simulink model "Com_hex2num_convert"  (R2017a)
settings: Solver=ode3  StartTime=0.0  StopTime=Inf  FixedStep=0.05  RelTol=1e-3  EnableMultiTasking=on
PostLoadFcn:
  | , if any(exist('dsrtsu_mdlpostloadfcn', 'file') == [2, 3, 6]), try dsrtsu_mdlpostloadfcn('Execute', bdroot); catch fprintf('Error in PostLoadFcn (dsrtsu_mdlpostloadfcn) for model "%s":\n %s\n', bdroot, lasterr); end, end,
undefined symbols (not defined in the file): serial
libraries: instrumentlib x2
settings Model: DSRTSU_INTERNAL_RTI_VER=500  DSRTSU_INTERNAL_RTI_TYPE=rti1401  DSRTSU_INTERNAL_RTIFPGA=90  Creator=Administrator  LastModifiedBy=Administrator
settings DataIOCC: SaveFormat=Array
settings OptimizationCC: BlockReduction=off  OptimizeBlockIOStorage=off  BufferReuse=off  GlobalBufferReuse=off  ExpressionFolding=off  LocalBlockOutputs=off  LifeSpan=inf
settings DebuggingCC: UnderspecifiedInitializationDetection=Classic  MergeDetectMultiDrivingBlocksExec=none  SolverPrmCheckMsg=warning  StateNameClashWarn=warning  SFUnexpectedBacktrackingDiag=warning  SFNoUnconditionalDefaultTransitionDiag=warning  SFExecutionAtInitializationDiag=none
settings HardwareCC: ProdBitPerPointer=32  ProdBitPerSizeT=32  ProdBitPerPtrDiffT=32  ProdLargestAtomicInteger=Integer  ProdEndianess=BigEndian  ProdWordSize=32  ProdHWDeviceType=Custom Processor->Custom  TargetIntDivRoundTo=Zero  TargetEndianess=BigEndian  TargetHWDeviceType=Custom Processor->Custom
settings ModelReferenceCC: PropagateSignalLabelsOutOfModel=off
settings SFSimCC: MATLABDynamicMemAlloc=off
settings RTWCC: SystemTargetFile=rti1005.tlc  MakeCommand=make_rti  TemplateMakefile=rti1005.tmf  Description=dSPACE DS1005 Hardware Platform
settings STFCustomTargetCC: ParMdlRefBuildCompliant=on  GRTInterface=off  SystemTargetFile=rti1005.tlc
settings GRTTargetCC: TargetLangStandard=C89/C90 (ANSI)  CompOptLevelCompliant=off  ConcurrentExecutionCompliant=off  CombineOutputUpdateFcns=off  MatFileLogging=off  CPPClassGenCompliant=off  UseToolchainInfoCompliant=off  ExtModeMexFile=noextcomm
settings ConfigComp: CovMetricSettings=dw  CovHtmlReporting=on  CovSaveCumulativeToWorkspaceVar=on  CovSaveSingleToWorkspaceVar=on  CovExternalEMLEnable=off  CovSFcnEnable=off

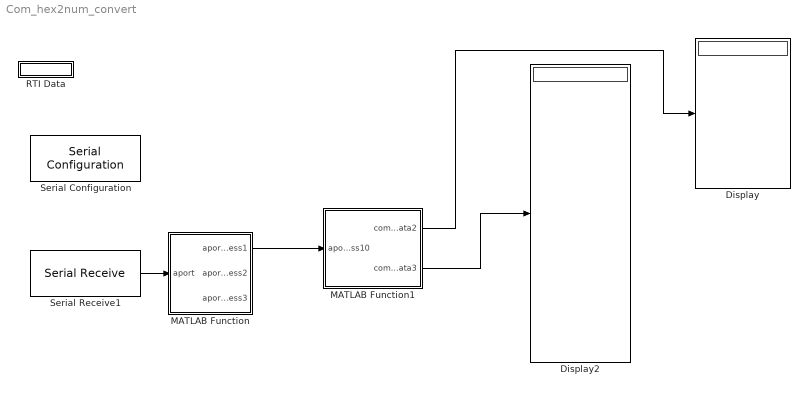
== system Com_hex2num_convert ==
  Display : Display
  Display2 : Display
  MATLAB Function : MATLAB Function  TreatAsAtomicUnit=on
  MATLAB Function1 : MATLAB Function  TreatAsAtomicUnit=on
  RTI Data : Subsystem  Tag=struct('RTIDataServer',struct('RTIDataServerVs','2','RTIModelDescription','struct(''main'',''Com_hex2num_convert'',''sub'',''Com_hex2num_convert'',''isMp'',0)'))  LoadFcn="if exist('rtidc'), try,  rtidc('DataHostBlockClbLoad', gcbh); catch, disp(['Warning: ''LoadFcn'' for RTI Data block failed: ' lasterr]); end, end,"  mask(RTI_DATA_HOST){}
      mask help:
      | RTI Data Block.
      | This block is used by RTI to store internal model-dependent data.
      | Please keep this block on the root level of the model. Deleting this block will result in data loss.
      |
      | NEVER DELETE OR COPY THIS BLOCK!
      settings: CopyFcn="if exist('rtidc'), try,  rtidc('DataHostBlockClbCopy', gcbh); catch, disp(['Warning: ''CopyFcn'' for RTI Data block failed: ' lasterr]); end, end,"  DeleteFcn="if exist('rtidc'), try,  rtidc('DataHostBlockClbDelete', gcbh); catch, disp(['Warning: ''DeleteFcn'' for RTI Data block failed: ' lasterr]); end, end,"  ModelCloseFcn="if exist('rtidc'), try,  rtidc('DataHostBlockClbModelClose', gcbh); catch, disp(['Warning: ''ModelCloseFcn'' for RTI Data block failed: ' lasterr]); end, end,"  PreSaveFcn="if exist('rtidc'), try,  rtidc('DataHostBlockClbPreSave', gcbh); catch, disp(['Warning: ''PreSaveFcn'' for RTI Data block failed: ' lasterr]); end, end,"  PostSaveFcn="if exist('rtidc'), try,  rtidc('DataHostBlockClbPostSave', gcbh); catch, disp(['Warning: ''PostSaveFcn'' for RTI Data block failed: ' lasterr]); end, end,"  NameChangeFcn="if exist('rtidc'), try,  rtidc('DataHostBlockClbNameChange', gcbh); catch, disp(['Warning: ''NameChangeFcn'' for RTI Data block failed: ' lasterr]); end, end,"
      mask Help:
      | RTI Data Block.
      | This block is used by RTI to store internal model-dependent data.
      | Please keep this block on the root level of the model. Deleting this block will result in data loss.
      | 
      | NEVER DELETE OR COPY THIS BLOCK!
      mask Display:
      | text(0.5, 0.5, 'RTI Data', 'HorizontalAlignment', 'center');
      | plot([1 0]);
  Serial Configuration : instrumentlib/Serial Configuration  Priority=-200000  ComPortMenu=<Please select a port...>  ComPort=COM4  ObjConstructor=serial('COM4');  BaudRate=115200  DataBits=8  Parity=none  StopBits=1  FlowControl=none  Timeout=10  ByteOrder=LittleEndian
  Serial Receive1 : instrumentlib/Serial Receive  ComPortMenu=<Please select a port...>  ComPort=COM4  ObjConstructor=serial('COM4');  Terminator=<none>  DataSize="[600    1]"  DataType=uint8  EnableBlockingMode=on  ActionDataUnavailable=Output last received value  CustomValue=0  SampleTime=0.05
  wires:
  Serial Receive1/1 -> MATLAB Function/1(aport)
  MATLAB Function/1(aport_mess1) -> MATLAB Function1/1(aport_mess10)
  MATLAB Function1/2(com_data3) -> Display2/1
  MATLAB Function1/1(com_data2) -> Display/1

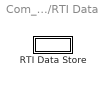
== system Com_hex2num_convert/RTI Data ==
  RTI Data Store : Subsystem  Tag=struct('private',struct('version',struct('dsVer',uint32(2),'dsVerCreation',uint32(2),'RTI',struct('ver','7.1','type','RTI1005')),'access',struct('type','Model','isPerm',1,'created',['10-Nov-2015 11:46:18'],'modified',['27-Sep-2017 17:37:50'],'location','')),'public',struct('main',struct('data',[]),'sub',struct('name','','data',[])))  mask(RTI_DATA_STORE){}
      mask help:
      | RTI Data Store Block. This block is used by RTI to store internal model dependent data. Deleting this block will result in data loss.
      |
      | NEVER DELETE, COPY, OR MODIFY THIS BLOCK!
      mask Help:
      | RTI Data Store Block. This block is used by RTI to store internal model dependent data. Deleting this block will result in data loss.
      | 
      | NEVER DELETE, COPY, OR MODIFY THIS BLOCK!
      mask Display: text(0.5, 0.5, ' ', 'HorizontalAlignment', 'center');

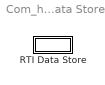
== system Com_hex2num_convert/RTI Data/RTI Data Store ==
  RTI Data Store : Subsystem  mask(RTI_DATA_STORE){}
      mask help:
      | RTI Data Store Block. This block is used by RTI to store internal model dependent data. Deleting this block will result in data loss.
      |
      | NEVER DELETE, COPY, OR MODIFY THIS BLOCK!
      mask Help:
      | RTI Data Store Block. This block is used by RTI to store internal model dependent data. Deleting this block will result in data loss.
      | 
      | NEVER DELETE, COPY, OR MODIFY THIS BLOCK!
      mask Display: text(0.5, 0.5, ' ', 'HorizontalAlignment', 'center');

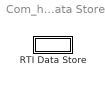
== system Com_hex2num_convert/RTI Data/RTI Data Store/RTI Data Store ==
  RTI Data Store : Subsystem  mask(RTI_DATA_STORE){}
      mask help:
      | RTI Data Store Block. This block is used by RTI to store internal model dependent data. Deleting this block will result in data loss.
      |
      | NEVER DELETE, COPY, OR MODIFY THIS BLOCK!
      mask Help:
      | RTI Data Store Block. This block is used by RTI to store internal model dependent data. Deleting this block will result in data loss.
      | 
      | NEVER DELETE, COPY, OR MODIFY THIS BLOCK!
      mask Display: text(0.5, 0.5, ' ', 'HorizontalAlignment', 'center');

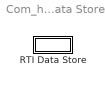
== system Com_hex2num_convert/RTI Data/RTI Data Store/RTI Data Store/RTI Data Store ==
  RTI Data Store : Subsystem  mask(RTI_DATA_STORE){}
      mask help:
      | RTI Data Store Block. This block is used by RTI to store internal model dependent data. Deleting this block will result in data loss.
      |
      | NEVER DELETE, COPY, OR MODIFY THIS BLOCK!
      mask Help:
      | RTI Data Store Block. This block is used by RTI to store internal model dependent data. Deleting this block will result in data loss.
      | 
      | NEVER DELETE, COPY, OR MODIFY THIS BLOCK!
      mask Display: text(0.5, 0.5, ' ', 'HorizontalAlignment', 'center');

== system Com_hex2num_convert/RTI Data/RTI Data Store/RTI Data Store/RTI Data Store/RTI Data Store ==

== matlab function Com_hex2num_convert/MATLAB Function1 ==
  data: aport_mess10 input; com_data2 output; com_data3 output
function [com_data2, com_data3]  = GNSS_data(aport_mess10)
com_data20=zeros(3,1);
com_data30=zeros(16,1);
for i=1
aport_mess1=aport_mess10(i,:);

com_01=aport_mess1(1:4);
com_01=fliplr(com_01);

com_02=(aport_mess1(5:8));  %time seconds
com_02=(dec2hex(fliplr(com_02)));
com_02=[com_02(1,:),com_02(2,:),com_02(3,:),com_02(4,:)];
com_02=hex2dec(com_02);

com_03=(aport_mess1(9:12));  %time microseconds
com_03=(dec2hex(fliplr(com_03)));
com_03=[com_03(1,:),com_03(2,:),com_03(3,:),com_03(4,:)];
com_03=hex2dec(com_03);


com_04=(aport_mess1(13:20));  %纬度  deg
com_04=(dec2hex(fliplr(com_04)));
com_040=[com_04(1,:),com_04(2,:),com_04(3,:),com_04(4,:),com_04(5,:),com_04(6,:),com_04(7,:),com_04(8,:)];
%hex2num(com_042)
com_0410=typecast(uint8((com_040)),'double');
com_041 = com_0410(1,1);
%com_041=com_041*180/pi;

com_05=(aport_mess1(21:28));  %经度 deg
com_05=(dec2hex(fliplr(com_05)));
com_05=[com_05(1,:),com_05(2,:),com_05(3,:),com_05(4,:),com_05(5,:),com_05(6,:),com_05(7,:),com_05(8,:)];
%com_051=[com_05(1,:),com_05(2,:),com_05(3,:),com_05(4,:)]
%com_051=hex2num(com_051);
%com_051=typecast((hex2dec(com_051)),'single')
%com_05=com_05*180/pi;
com_051=0;

com_06=(aport_mess1(29:36));  %高度 m
com_06=(dec2hex(fliplr(com_06)));
com_06=[com_06(1,:),com_06(2,:),com_06(3,:),com_06(4,:),com_06(5,:),com_06(6,:),com_06(7,:),com_06(8,:)];
%com_061=[com_06(1,:),com_06(2,:),com_06(3,:),com_06(4,:)]
%com_061=[com_06(5,:),com_06(6,:),com_06(7,:),com_06(8,:)]
%com_061=hex2num(com_061);
%com_061=typecast((hex2dec(com_061)),'single')
com_061=0;

com_07=(aport_mess1(37:40));  %北向速度 （m/s）
com_07=(dec2hex(fliplr(com_07)));
com_07=[com_07(1,:),com_07(2,:),com_07(3,:),com_07(4,:)];
com_07=typecast(uint32(hex2dec(com_07)),'single');

com_08=(aport_mess1(41:44));  %东向速度 （m/s）
com_08=(dec2hex(fliplr(com_08)));
com_08=[com_08(1,:),com_08(2,:),com_08(3,:),com_08(4,:)];
com_08=typecast(uint32(hex2dec(com_08)),'single');

com_09=(aport_mess1(45:48));  %地向速度 （m/s）
com_09=(dec2hex(fliplr(com_09)));
com_09=[com_09(1,:),com_09(2,:),com_09(3,:),com_09(4,:)];
com_09=typecast(uint32(hex2dec(com_09)),'single');

com_10=(aport_mess1(49:52));  % 载体加速度 X（m/s/s）
com_10=(dec2hex(fliplr(com_10)));
com_10=[com_10(1,:),com_10(2,:),com_10(3,:),com_10(4,:)];
com_10=typecast(uint32(hex2dec(com_10)),'single');

com_11=(aport_mess1(53:56));  % 载体加速度 Y（m/s/s）
com_11=(dec2hex(fliplr(com_11)));
com_11=[com_11(1,:),com_11(2,:),com_11(3,:),com_11(4,:)];
com_11=typecast(uint32(hex2dec(com_11)),'single');

com_12=(aport_mess1(57:60));  % 载体加速度 Z（m/s/s）
com_12=(dec2hex(fliplr(com_12)));
com_12=[com_12(1,:),com_12(2,:),com_12(3,:),com_12(4,:)];
com_12=typecast(uint32(hex2dec(com_12)),'single');

com_13=(aport_mess1(61:64));  % % 重力加速度 （g）
com_13=(dec2hex(fliplr(com_13)));
com_13=[com_13(1,:),com_13(2,:),com_13(3,:),com_13(4,:)];
com_13=typecast(uint32(hex2dec(com_13)),'single');

com_14=(aport_mess1(65:68));  %横滚 （roll  rad）
com_14=(dec2hex(fliplr(com_14)));
com_14=[com_14(1,:),com_14(2,:),com_14(3,:),com_14(4,:)];
com_14=typecast(uint32(hex2dec(com_14)),'single')*180/pi;  % （deg/s）

com_15=(aport_mess1(69:72));   %俯仰 （roll  rad）
com_15=(dec2hex(fliplr(com_15)));
com_15=[com_15(1,:),com_15(2,:),com_15(3,:),com_15(4,:)];
com_15=typecast(uint32(hex2dec(com_15)),'single')*180/pi;  % （deg/s）

com_16=(aport_mess1(73:76));   %航向 （roll  rad）
com_16=(dec2hex(fliplr(com_16)));
com_16=[com_16(1,:),com_16(2,:),com_16(3,:),com_16(4,:)];
com_16=typecast(uint32(hex2dec(com_16)),'single')*180/pi;  % （deg/s）

com_17=(aport_mess1(77:80));  %角速度 X （rad/s）
com_17=(dec2hex(fliplr(com_17)));
com_17=[com_17(1,:),com_17(2,:),com_17(3,:),com_17(4,:)];
com_17=typecast(uint32(hex2dec(com_17)),'single')*180/pi;  %角速度 X （deg/s）

com_18=(aport_mess1(81:84));  %角速度 Y （rad/s）
com_18=(dec2hex(fliplr(com_18)));
com_18=[com_18(1,:),com_18(2,:),com_18(3,:),com_18(4,:)];
com_18=typecast(uint32(hex2dec(com_18)),'single')*180/pi;  %角速度 Y （deg/s）

com_19=(aport_mess1(85:88));  %角速度 Z （rad/s）
com_19=(dec2hex(fliplr(com_19)));
com_19=[com_19(1,:),com_19(2,:),com_19(3,:),com_19(4,:)];
com_19=typecast(uint32(hex2dec(com_19)),'single')*180/pi;  %角速度 Z （deg/s）

com_20=(aport_mess1(89:92));  %纬度标准差（m）
com_20=(dec2hex(fliplr(com_20)));
com_20=[com_20(1,:),com_20(2,:),com_20(3,:),com_20(4,:)];
com_20=typecast(uint32(hex2dec(com_20)),'single');

com_21=(aport_mess1(93:96));  %经度标准差（m）
com_21=(dec2hex(fliplr(com_21)));
com_21=[com_21(1,:),com_21(2,:),com_21(3,:),com_21(4,:)];
com_21=typecast(uint32(hex2dec(com_21)),'single');

com_22=(aport_mess1(97:100));  %高度标准差（m）
com_22=(dec2hex(fliplr(com_22)));
com_22=[com_22(1,:),com_22(2,:),com_22(3,:),com_22(4,:)];
com_22= typecast(uint32(hex2dec(com_22)),'single');

com_data1=[com_01,com_02,com_03]';     %% time 
com_data20(:,i)=[com_041,com_051,com_061]';    
com_data30(:,i)=[com_07,com_08,com_09,...
          com_10,com_11,com_12,com_13,com_14,com_15,com_16,com_17,com_18,com_19,com_20,com_21,com_22]';  %% 
end
com_data2=com_data20;
com_data3=com_data30;

== matlab function Com_hex2num_convert/MATLAB Function ==
  data: aport input; aport_mess1 output; aport_mess2 output; aport_mess3 output
function [ aport_mess1,aport_mess2,aport_mess3] = LRC_my(aport)
%global string1
string1=zeros(117,15);
string2=zeros(127,15);
aport_hex0=dec2hex(aport);
aport_hex=(aport);
n=1;
for m=1:length(aport)-4
    
        aport_h1=aport_hex(m);
        aport_h2=aport_hex(m+1:m+4);
        aport_h10=dec2hex(aport_h1);
        aport_h20=dec2hex(aport_h2);
        StringIn=aport_h20;
    out=StringIn;
    mes=StringIn;
    decmes = hex2dec(mes);      % convert to dec
    sumdec = sum(decmes);       %sum the decimal values
    hexsum = dec2hex(sumdec,4); % generate a 4 digit hex number
    binsum = dec2bin(sumdec,8); % genearte 8bit binary number
    
    % Handle the number being large
    if length(binsum) > 8
        binsum = binsum(length(binsum)-7:length(binsum));
    end
        empbin = ['00000000'];  % start with an empty binary number
        firstfind = 0;
    for i = 1:length(binsum)
        if binsum(end+1-i) == '0'
            if firstfind == '0'
                %leave as 0
            elseif firstfind == 1
               empbin(end+1-i) = '1';    %swap a 1 for 0
            end
        elseif binsum(end+1-i) == '1'
            if firstfind == 0
                empbin(end+1-i) = '1';
                firstfind = 1;
            elseif firstfind == 1
                empbin(end+1-i) = '0';
            end
        else
                disp('Error in LRC calculation')
        end
    end

    CalcLRC0 = dec2hex(bin2dec(empbin),2); % LRC calculated by the program 16进制
    (aport_h10);  %% 16进制

    aport_h1;  %% 10进制
    CalcLRC=hex2dec(CalcLRC0) ;%% 10进制  用10进制对比，不然 08 十六进制 仅存为8 ，判断相等时出问题  
    
    Lout = length(out);
   % out(Lout+1:Lout+2) = CalcLRC  %% 原文
   out;
   m;
   aport_h20(1,:);
  if strcmpi(aport_h20(1,:),'14')&& aport_h1==CalcLRC  %%改进
    %  pause
     % length(aport_hex(m+5:m+121))
      if length(aport)-(m+121) >= 122
   % string = [CalcLRC;out]
    report = 1;
   string10=aport_hex(m+5:m+121);
   string20=aport_hex(m:m+126);
   string1(:,n)=string10;
   string2(:,n)=string20;
     n=n+1;
    % pause
      else 
     
   string1(:,n)=string1(:,n-1);
   string2(:,n)=string2(:,n-1);        
      
  end
  end
end
n;



%aport_mess1=(string1(:,1))' ;  % 行向量输出
aport_mess1=(string1)' ; % 行向量输出
aport_mess2=(string2)';

aport_mess3=(string1(:,1))';
